simulink model "Task1_b_2"  (R2024b)
settings: Solver=VariableStepAuto  StartTime=0.0  StopTime=10.0  RelTol=1e-3
settings Model: Creator=max  LastModifiedBy=max

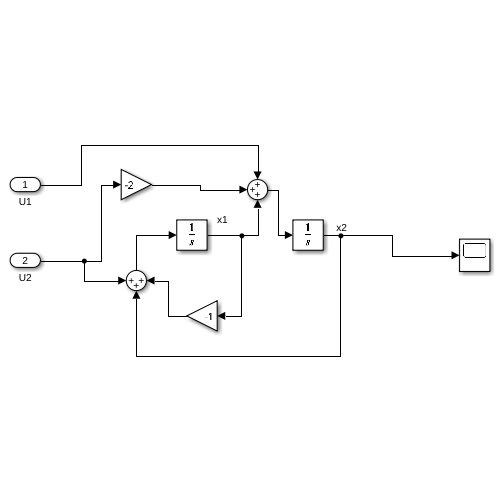
[thumbnail: Simulink's stored preview of the top-level diagram]
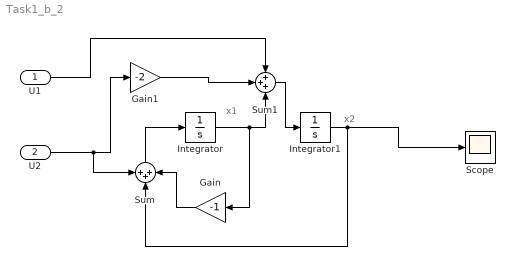
== system Task1_b_2 ==
  note: x1
  note: x2
  U1 : Inport
  U2 : Inport  Port=2
  Gain : Gain  Gain=-1
  Gain1 : Gain  Gain=-2
  Integrator : Integrator
  Integrator1 : Integrator
  Scope : Scope
  Sum : Sum  Inputs=+++
  Sum1 : Sum  Inputs=+++
  wires:
  Integrator1/1 -> Sum/2, Scope/1
  Integrator/1 -> Sum1/3, Gain/1
  Gain/1 -> Sum/3
  U2/1 -> Gain1/1, Sum/1
  Sum/1 -> Integrator/1
  U1/1 -> Sum1/1
  Gain1/1 -> Sum1/2
  Sum1/1 -> Integrator1/1
